simulink model "mcb_pmsm_foc_sensorless_hvkit_f28069m"  (R2021b)
settings: Solver=FixedStepDiscrete  StartTime=0.0  StopTime=8  RelTol=1e-3  EnableMultiTasking=on
InitFcn:
  | mcb_pmsm_foc_sensorless_hvkit_f28069m_datascript;
values from neighbouring files (symbols this model uses):
  acceleration = 20000/PU_System.N_base    [mcb_pmsm_foc_dual_f28379d_datascript.m]    (also in mcb_pmsm_foc_sensorless_dyno_f28379d_datascript.m = 20000/PU_System_motor1.N_base; mcb_pmsm_foc_sensorless_f280049C_datascript.m; mcb_pmsm_foc_sensorless_f28027LaunchPad_data.m; mcb_pmsm_foc_sensorless_f28035_datascript.m)
  inverter = mcb_SetInverterParameters('BoostXL-DRV8305')    [mcb_pmsm_foc_dual_f28379d_data.m]    (also in mcb_pmsm_foc_dual_f28379d_datascript.m; mcb_pmsm_foc_f280049C_data.m; mcb_pmsm_foc_f28335_data.m = mcb_SetInverterParameters('DRV8312-C2-KIT'); mcb_pmsm_foc_hall_f28035_data.m = mcb_SetInverterParameters('DRV8312-C2-KIT'))
  PI_params = mcb.internal.SetControllerParameters(pmsm,inverter,PU_System,T_pwm,2*Ts,Ts_speed)    [mcb_pmsm_foc_dual_f28379d_data.m]    (also in mcb_pmsm_foc_dual_f28379d_datascript.m; mcb_pmsm_foc_f280049C_data.m = mcb.internal.SetControllerParameters(pmsm,inverter,PU_System; mcb_pmsm_foc_f28335_data.m = mcb.internal.SetControllerParameters(pmsm,inverter,PU_System; mcb_pmsm_foc_hall_f28035_data.m = mcb.internal.SetControllerParameters(pmsm,inverter,PU_System)
  pmsm = struct    [c28335_pmsmfoc_data.m]    (also in mcb_pmsm_foc_dual_f28379d_data.m = mcb_SetPMSMMotorParameters('Teknic2310P'); mcb_pmsm_foc_dual_f28379d_datascript.m = mcb_SetPMSMMotorParameters('Teknic2310P'); mcb_pmsm_foc_f280049C_data.m = mcb_SetPMSMMotorParameters('BLY171D'); mcb_pmsm_foc_f28335_data.m = mcb_SetPMSMMotorParameters('BLY171D'))
  PWM_frequency = 20e3    (= 20000)    [c28027pmsmfoc_data.m]    (also in c28035pmsmfoc_data.m; c28035pmsmfoc_data_cla.m = 12000; c28069pmsmfoc_data.m; mcb_c2000_open_loop_control_data.m = eval(get_param([bdroot '/Open Loop Control/Parameters/PWM Fr)
  Speed_openLoop_PU = 0.1    [mcb_pmsm_foc_dual_f28379d_data.m]    (also in mcb_pmsm_foc_dual_f28379d_datascript.m; mcb_pmsm_foc_sensorless_dyno_f28379d_data.m; mcb_pmsm_foc_sensorless_dyno_f28379d_datascript.m; mcb_pmsm_foc_sensorless_f280049C_data.m)
  T_Ref_openLoop = 1    [mcb_pmsm_foc_dual_f28379d_data.m]    (also in mcb_pmsm_foc_dual_f28379d_datascript.m; mcb_pmsm_foc_sensorless_dyno_f28379d_data.m; mcb_pmsm_foc_sensorless_dyno_f28379d_datascript.m; mcb_pmsm_foc_sensorless_f280049C_data.m)
  target = mcb_SetProcessorDetails('F28379D',PWM_frequency)    [mcb_pmsm_foc_dual_f28379d_data.m]    (also in mcb_pmsm_foc_dual_f28379d_datascript.m; mcb_pmsm_foc_f280049C_data.m = mcb_SetProcessorDetails('F280049C',PWM_frequency); mcb_pmsm_foc_f28335_data.m = mcb_SetProcessorDetails('F28335',PWM_frequency); mcb_pmsm_foc_hall_f28035_data.m = mcb_SetProcessorDetails('F28035',PWM_frequency))
  Ts_motor = T_pwm/2    (= 2.5e-05)    [mcb_pmsm_foc_dual_f28379d_data.m]    (also in mcb_pmsm_foc_dual_f28379d_datascript.m; mcb_pmsm_foc_f280049C_data.m; mcb_pmsm_foc_f28335_data.m; mcb_pmsm_foc_hall_f28035_data.m)
  Ts_simulink = T_pwm/2    (= 2.5e-05)    [mcb_pmsm_foc_dual_f28379d_data.m]    (also in mcb_pmsm_foc_dual_f28379d_datascript.m; mcb_pmsm_foc_f280049C_data.m; mcb_pmsm_foc_f28335_data.m; mcb_pmsm_foc_hall_f28035_data.m)
  Ts_speed = 20*Ts    (= 0.001)    [mcb_pmsm_foc_dual_f28379d_data.m]    (also in mcb_pmsm_foc_dual_f28379d_datascript.m; mcb_pmsm_foc_f280049C_data.m = 0.0005; mcb_pmsm_foc_f28335_data.m = 0.0005; mcb_pmsm_foc_hall_f28035_data.m = 0.0005)
undefined symbols (not defined in the file or in its folder): Down, GPTRIP1SEL, GPTRIP2SEL, TZ1, TZ2, Up
libraries: c2802xlib x5, c2806xlib x3, demo_controls x1, mcbplantlib x1, mcbcontrolslib x1, mcbpositiondecoderlib x1, autolibpmsmexterior x1
settings Model: ExtModeTrigDuration=8  Creator=The MathWorks, Inc.  LastModifiedBy=The MathWorks, Inc.
settings SolverCC: AlgebraicLoopSolver=TrustRegion
settings DataIOCC: LimitDataPoints=on  SaveFormat=Array  SaveOutput=off  SaveTime=off  ReturnWorkspaceOutputs=off
settings OptimizationCC: DefaultParameterBehavior=Inlined  OptimizeBlockIOStorage=off  BufferReuse=off  GlobalBufferReuse=off  ExpressionFolding=off  ExpressionDepthLimit=2147483647  LocalBlockOutputs=off  InitFltsAndDblsToZero=on  NoFixptDivByZeroProtection=on  EfficientFloat2IntCast=on  EfficientMapNaN2IntZero=off  LifeSpan=inf  MaxStackSize=768  OptimizeDataStoreBuffers=off  BusAssignmentInplaceUpdate=off  EfficientTunableParamExpr=on
settings DebuggingCC: ReadBeforeWriteMsg=DisableAll  WriteAfterWriteMsg=DisableAll  WriteAfterReadMsg=DisableAll  AlgebraicLoopMsg=error  ArtificialAlgebraicLoopMsg=error  CheckSSInitialOutputMsg=off  MergeDetectMultiDrivingBlocksExec=none  SignalResolutionControl=TryResolveAllWithWarning  SolverPrmCheckMsg=warning  InheritedTsInSrcMsg=none  MultiTaskDSMMsg=none  MultiTaskCondExecSysMsg=none  TasksWithSamePriorityMsg=none  SigSpecEnsureSampleTimeMsg=none  IntegerOverflowMsg=none  ParameterPrecisionLossMsg=none  FcnCallInpInsideContextMsg=warning  AllowSymbolicDim=off  StateNameClashWarn=warning  SFUnexpectedBacktrackingDiag=warning  SFNoUnconditionalDefaultTransitionDiag=warning  SFExecutionAtInitializationDiag=none  SFMachineParentedDataDiag=warning  IntegerSaturationMsg=none  ArithmeticOperatorsInVariantConditions=warning
settings HardwareCC: ProdBitPerChar=16  ProdBitPerInt=16  ProdBitPerPointer=32  ProdBitPerSizeT=32  ProdBitPerPtrDiffT=32  ProdLargestAtomicInteger=Integer  ProdLargestAtomicFloat=None  ProdWordSize=16  ProdLongLongMode=on  ProdHWDeviceType=Texas Instruments->C2000  TargetBitPerChar=16  TargetBitPerInt=16  TargetBitPerPointer=16  TargetLargestAtomicInteger=Integer  TargetIntDivRoundTo=Zero  TargetEndianess=LittleEndian  TargetWordSize=16  TargetHWDeviceType=Texas Instruments->C2000
settings ModelReferenceCC: PropagateSignalLabelsOutOfModel=off
settings SFSimCC: SimUseLocalCustomCode=off  MATLABDynamicMemAlloc=off
settings RTWCC: Description=Embedded Coder  SystemTargetFile=ert.tlc  HardwareBoard=TI Piccolo F2806x  TemplateMakefile=ert_default_tmf  PostCodeGenCommand=; codertarget.postCodeGenHookCommand(h)  GenerateReport=on  RTWUseLocalCustomCode=off  Toolchain=Texas Instruments Code Composer Studio (C2000)  BuildConfiguration=Faster Runs  IncludeHyperlinkInReport=on  LaunchReport=on  GenerateTraceInfo=on  GenerateTraceReport=on  GenerateTraceReportSl=on  GenerateTraceReportSf=on  GenerateTraceReportEml=on
settings CodeAppCC: IgnoreCustomStorageClasses=off  CustomSymbolStrType=$N$R$M  StateflowObjectComments=on  InternalIdentifier=Classic
settings ERTTargetCC: TargetFcnLib=ansi_tfl_tmw_new.mat  CodeReplacementLibrary=TI C28x  MultiwordLength=2048  ParMdlRefBuildCompliant=off  CompOptLevelCompliant=off  ConcurrentExecutionCompliant=off  CPPClassGenCompliant=off  ExtModeStaticAllocSize=2048  ExtModeMexFile=TIC2000ExternalModeOpen  ExtModeIntrfLevel=Level2 - Open  InlinedParameterPlacement=NonHierarchical  ConvertIfToSwitch=off  SuppressUnreachableDefaultCases=off  MemSecPackage=tic2000demospkg
settings ConfigComp: CovMetricSettings=dw  CovSaveCumulativeToWorkspaceVar=on  CovSaveSingleToWorkspaceVar=on  CovExternalEMLEnable=off  CovSFcnEnable=off

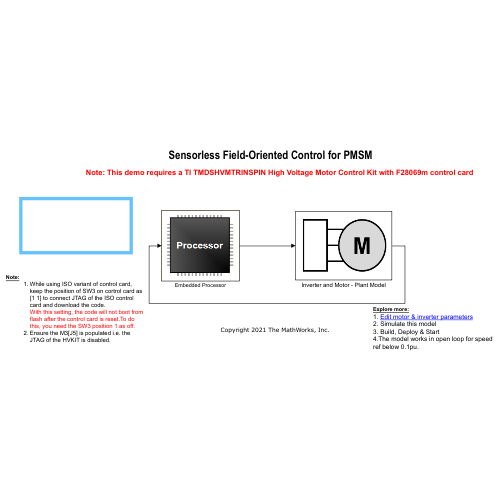
[thumbnail: Simulink's stored preview of the top-level diagram]
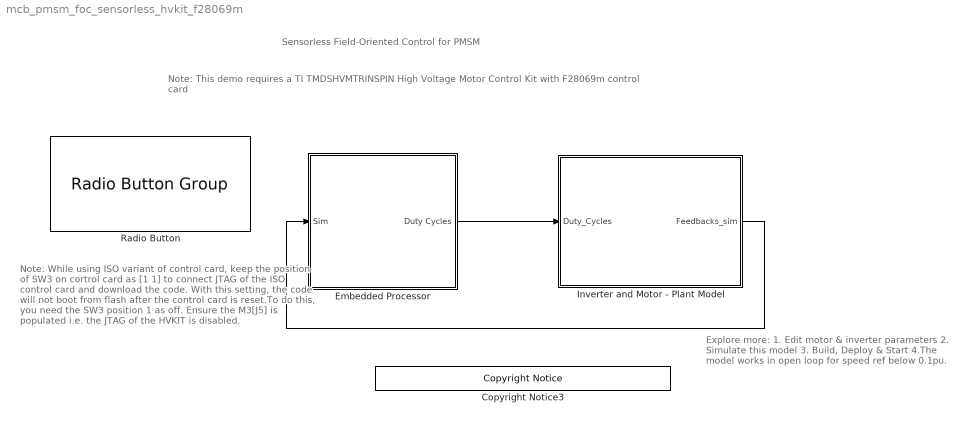
== system mcb_pmsm_foc_sensorless_hvkit_f28069m ==
  note: Sensorless Field-Oriented Control for PMSM
  note: Explore more:
      | 1. Edit motor & inverter parameters
      | 2. Simulate this model
      | 3. Build, Deploy & Start
      | 4.The model works in open loop for speed ref below 0.1pu.
  note: Note: This demo requires a TI TMDSHVMTRINSPIN High Voltage Motor Control Kit with F28069m control card
  note: Note:
      | While using ISO variant of control card, keep the position of SW3 on cortrol card as [1 1] to connect JTAG of the ISO control card and download the code.
      | With this setting, the code will not boot from flash after the control card is reset.To do this, you need the SW3 position 1 as off.
      | Ensure the M3[J5] is populated i.e. the JTAG of the HVKIT is disabled.
  Copyright Notice3 : demo_controls/Copyright Notice  year=2021  prod=tic2000
      settings: SourceProductBaseCode=ME
  Embedded Processor : Subsystem
      mask Display: image('mcb_pmsmfoc_processor.png')
  Inverter and Motor - Plant Model : Subsystem
      mask Display: image('mcb_pmsmfoc_motor.png')
  Radio Button : RadioButtonGroup  LabelPosition=Hide  SelectedLabel=Flux observer  ButtonGroupName=Postion Estimator
      settings: Values={{'Sliding mode observer', 'Flux observer'}, [0 1]}
  wires:
  Embedded Processor/1(Duty Cycles) -> Inverter and Motor - Plant Model/1(Duty_Cycles)
  Inverter and Motor - Plant Model/1(Feedbacks_sim) -> Embedded Processor/1(Sim)

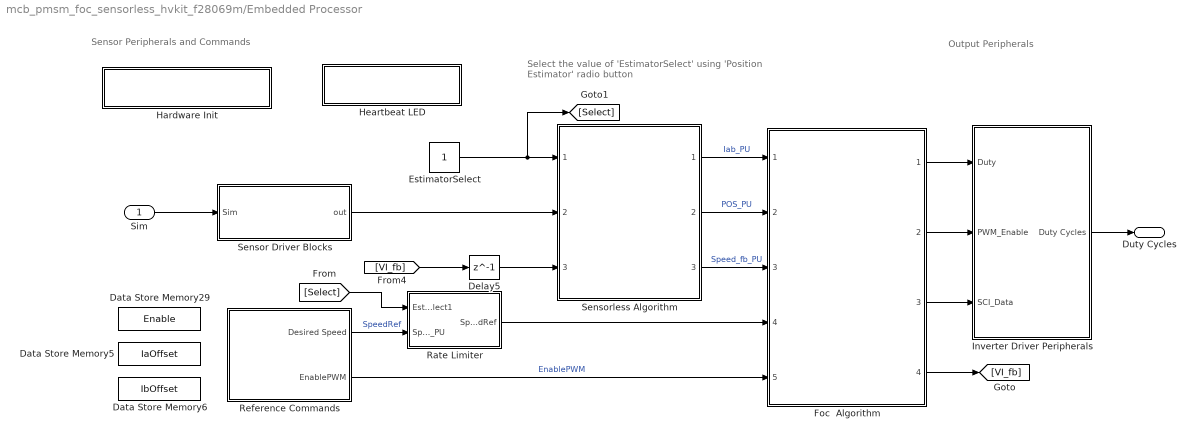
== system mcb_pmsm_foc_sensorless_hvkit_f28069m/Embedded Processor ==
  note: Output Peripherals
  note: Sensor Peripherals and Commands
  note: Select the value of 'EstimatorSelect' using 'Position Estimator' radio button
  Sim : Inport
  Data Store Memory29 : DataStoreMemory  DataStoreName=Enable  ReadBeforeWriteMsg=warning  WriteAfterWriteMsg=warning  WriteAfterReadMsg=warning  InitialValue=1  ShowAdditionalParam=off  OutDataTypeStr=boolean
  Data Store Memory5 : DataStoreMemory  DataStoreName=IaOffset  InitialValue=inverter.CtSensAOffset  ShowAdditionalParam=off  OutDataTypeStr=uint16
  Data Store Memory6 : DataStoreMemory  DataStoreName=IbOffset  InitialValue=inverter.CtSensBOffset  ShowAdditionalParam=off  OutDataTypeStr=uint16
  Delay5 : Delay  DelayLength=1
  EstimatorSelect : Constant
  Foc  Algorithm : Subsystem  ReferencedSubsystem=foc_sensorless_algorithm
  Hardware Init : Subsystem  TreatAsAtomicUnit=on
  Heartbeat LED : Subsystem  TreatAsAtomicUnit=on
  Inverter Driver Peripherals : Subsystem  TreatAsAtomicUnit=on
      settings: RTWSystemCode=Nonreusable function
  Rate Limiter : Subsystem  SystemSampleTime=Ts_speed
  Reference Commands : Subsystem  SystemSampleTime=1e-3
  Sensor Driver Blocks : Subsystem  Variant=on  VariantControlMode=sim codegen switching
  Sensorless Algorithm : Subsystem  TreatAsAtomicUnit=on  ReferencedSubsystem=sensorless_algorithm
      settings: RTWSystemCode=Nonreusable function
  Duty Cycles : Outport
  wires:
  Reference Commands/1(Desired Speed) -> Rate Limiter/2(Speed_Ref_PU)  "SpeedRef"
  Inverter Driver Peripherals/1(Duty Cycles) -> Duty Cycles/1
  Reference Commands/2(EnablePWM) -> Foc  Algorithm/5  "EnablePWM"
  Foc  Algorithm/4 -> [VI_fb]
  [VI_fb] -> Delay5/1
  Foc  Algorithm/3 -> Inverter Driver Peripherals/3(SCI_Data)
  Sensorless Algorithm/1 -> Foc  Algorithm/1  "Iab_PU"
  Sensorless Algorithm/2 -> Foc  Algorithm/2  "POS_PU"
  Sensorless Algorithm/3 -> Foc  Algorithm/3  "Speed_fb_PU"
  Foc  Algorithm/2 -> Inverter Driver Peripherals/2(PWM_Enable)
  Foc  Algorithm/1 -> Inverter Driver Peripherals/1(Duty)
  Sim/1 -> Sensor Driver Blocks/1(Sim)
  Delay5/1 -> Sensorless Algorithm/3
  Sensor Driver Blocks/1(out) -> Sensorless Algorithm/2
  Rate Limiter/1(SpeedRef) -> Foc  Algorithm/4
  EstimatorSelect/1 -> [Select], Sensorless Algorithm/1
  [Select] -> Rate Limiter/1(EstimatorSelect1)

== system mcb_pmsm_foc_sensorless_hvkit_f28069m/Inverter and Motor - Plant Model ==
  Duty_Cycles : Inport
  Inverter and Motor - Plant Model : Subsystem
  RT3 : RateTransition  Deterministic=off
  Rate Transition2 : RateTransition  Deterministic=off  OutPortSampleTime=Ts
  Feedbacks_sim : Outport  VectorParamsAs1DForOutWhenUnconnected=off
  wires:
  RT3/1 -> Inverter and Motor - Plant Model/1(Duty_Cycles)
  Inverter and Motor - Plant Model/1(Feedbacks_sim) -> Rate Transition2/1
  Duty_Cycles/1 -> RT3/1
  Rate Transition2/1 -> Feedbacks_sim/1

== system mcb_pmsm_foc_sensorless_hvkit_f28069m/Embedded Processor/Hardware Init ==
  Event Listener : EventListener  DisableCoverage=on  EventName=reset
  Offset Calculation : Subsystem  Variant=on  VariantControlMode=sim codegen switching  VariantControl=Choice

== system mcb_pmsm_foc_sensorless_hvkit_f28069m/Embedded Processor/Heartbeat LED ==
  note: Heartbeat LED 1HZ
  LED BLINK : Subsystem  Variant=on  VariantControlMode=sim codegen switching  VariantControl=Choice
  RED_LED : Constant  OutDataTypeStr=uint16  SampleTime=0.5
  wires:
  RED_LED/1 -> LED BLINK/1(In1)

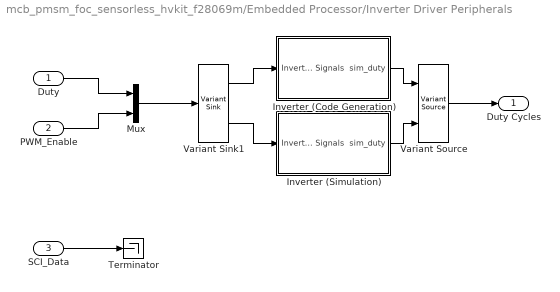
== system mcb_pmsm_foc_sensorless_hvkit_f28069m/Embedded Processor/Inverter Driver Peripherals ==
  Duty : Inport
  PWM_Enable : Inport  Port=2
  SCI_Data : Inport  Port=3
  Inverter (Code Generation) : Subsystem  VariantControl=Choice
  Inverter (Simulation) : Subsystem  VariantControl=(sim)
  Mux : Mux  Inputs=2
  Terminator : Terminator
  Variant Sink1 : VariantSink  VariantControlMode=sim codegen switching
  Variant Source : VariantSource  VariantControlMode=sim codegen switching
  Duty Cycles : Outport  InitialOutput=0  VectorParamsAs1DForOutWhenUnconnected=off
  wires:
  Variant Source/1 -> Duty Cycles/1
  PWM_Enable/1 -> Mux/2
  Duty/1 -> Mux/1
  Mux/1 -> Variant Sink1/1
  Variant Sink1/1 -> Inverter (Code Generation)/1(Inverter Signals)
  Variant Sink1/2 -> Inverter (Simulation)/1(Inverter Signals)
  Inverter (Code Generation)/1(sim_duty) -> Variant Source/1
  Inverter (Simulation)/1(sim_duty) -> Variant Source/2
  SCI_Data/1 -> Terminator/1

== system mcb_pmsm_foc_sensorless_hvkit_f28069m/Embedded Processor/Rate Limiter ==
  EstimatorSelect1 : Inport
  Speed_Ref_PU : Inport  Port=2
  RT3 : RateTransition  Deterministic=off  OutPortSampleTime=Ts_speed
  Slew Rate : Subsystem  TreatAsAtomicUnit=on  SystemSampleTime=Ts_speed
  SpeedRef : Outport
  wires:
  Speed_Ref_PU/1 -> RT3/1
  EstimatorSelect1/1 -> Slew Rate/1(In1)
  RT3/1 -> Slew Rate/2(Speed_Ref)
  Slew Rate/1(Out1) -> SpeedRef/1

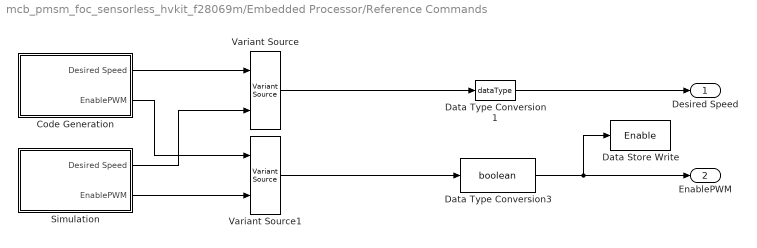
== system mcb_pmsm_foc_sensorless_hvkit_f28069m/Embedded Processor/Reference Commands ==
  Code Generation : Subsystem
  Data Store Write : DataStoreWrite  DataStoreName=Enable  IndexOptions=Index vector (dialog)  Indices=1  OutputSizes=1
  Data Type Conversion1 : DataTypeConversion  OutDataTypeStr=dataType  RndMeth=Simplest
  Data Type Conversion3 : DataTypeConversion  OutDataTypeStr=boolean  RndMeth=Simplest
  Simulation : Subsystem
  Variant Source : VariantSource  VariantControlMode=sim codegen switching
  Variant Source1 : VariantSource  VariantControlMode=sim codegen switching
  Desired Speed : Outport  VectorParamsAs1DForOutWhenUnconnected=off
  EnablePWM : Outport  Port=2
  wires:
  Data Type Conversion3/1 -> Data Store Write/1, EnablePWM/1
  Data Type Conversion1/1 -> Desired Speed/1
  Simulation/2(EnablePWM) -> Variant Source1/2
  Code Generation/2(EnablePWM) -> Variant Source1/1
  Simulation/1(Desired Speed) -> Variant Source/2
  Variant Source1/1 -> Data Type Conversion3/1
  Code Generation/1(Desired Speed) -> Variant Source/1
  Variant Source/1 -> Data Type Conversion1/1

== system mcb_pmsm_foc_sensorless_hvkit_f28069m/Embedded Processor/Sensor Driver Blocks ==
  Sim : Inport
  Sensor Driver Blocks (codegen) : Subsystem  TreatAsAtomicUnit=on  VariantControl=(codegen)
      settings: RTWSystemCode=Nonreusable function
  Sensor Driver Blocks (sim) : Subsystem  VariantControl=(sim)
  out : Outport

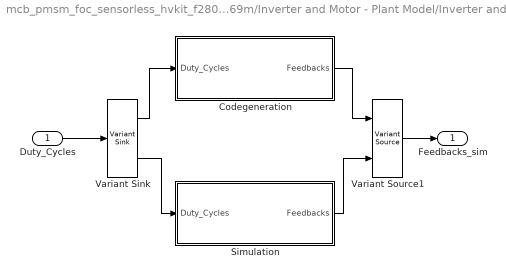
== system mcb_pmsm_foc_sensorless_hvkit_f28069m/Inverter and Motor - Plant Model/Inverter and Motor - Plant Model ==
  Duty_Cycles : Inport
  Codegeneration : Subsystem
  Simulation : Subsystem
  Variant Sink : VariantSink  VariantControlMode=sim codegen switching
  Variant Source1 : VariantSource  VariantControlMode=sim codegen switching
  Feedbacks_sim : Outport  VectorParamsAs1DForOutWhenUnconnected=off
  wires:
  Duty_Cycles/1 -> Variant Sink/1
  Simulation/1(Feedbacks) -> Variant Source1/2
  Variant Sink/2 -> Simulation/1(Duty_Cycles)
  Variant Source1/1 -> Feedbacks_sim/1
  Variant Sink/1 -> Codegeneration/1(Duty_Cycles)
  Codegeneration/1(Feedbacks) -> Variant Source1/1

== system mcb_pmsm_foc_sensorless_hvkit_f28069m/Embedded Processor/Hardware Init/Offset Calculation ==
  Code Generation : Subsystem  VariantControl=(codegen)
  Simulation : Subsystem  VariantControl=(sim)

== system mcb_pmsm_foc_sensorless_hvkit_f28069m/Embedded Processor/Heartbeat LED/LED BLINK ==
  In1 : Inport
  Code generation : Subsystem  VariantControl=(codegen)
  Simulation : Subsystem  VariantControl=(sim)

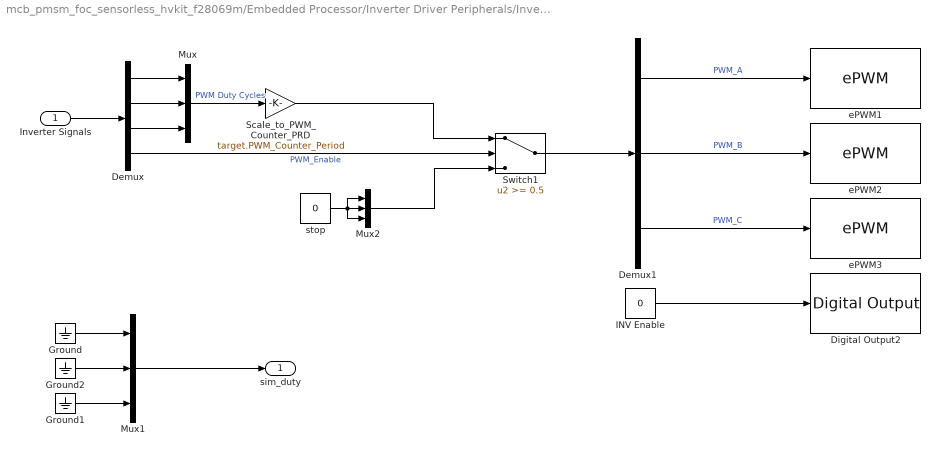
== system mcb_pmsm_foc_sensorless_hvkit_f28069m/Embedded Processor/Inverter Driver Peripherals/Inverter (Code Generation) ==
  Inverter Signals : Inport
  Demux : Demux
  Demux1 : Demux  Outputs=3
  Digital Output2 : c2806xlib/Digital Output  GPIO_Number=GPIO8~GPIO15  GPIO_Bit0=off  GPIO_BIT0_Toggle=off  GPIO_Bit1=off  GPIO_BIT1_Toggle=off  GPIO_Bit2=off  GPIO_BIT2_Toggle=off  GPIO_Bit3=off  GPIO_BIT3_Toggle=off  GPIO_Bit4=off  GPIO_BIT4_Toggle=off  GPIO_Bit5=off  GPIO_BIT5_Toggle=off  GPIO_Bit6=off  GPIO_BIT6_Toggle=off  GPIO_Bit7=on  GPIO_BIT7_Toggle=off
      settings: SourceProductBaseCode=TIC2000
  Ground : Ground
  Ground1 : Ground
  Ground2 : Ground
  INV Enable : Constant  Value=0  OutDataTypeStr=uint16
  Mux : Mux  Inputs=3
  Mux1 : Mux  Inputs=3
  Mux2 : Mux  Inputs=3
  Scale_to_PWM_Counter_PRD : Gain  Gain=target.PWM_Counter_Period  OutDataTypeStr=uint16  RndMeth=Simplest
  Switch1 : Switch  Threshold=0.5
  ePWM1 : c2802xlib/ePWM  PwmType=C2000  useModule=ePWM1  ePWMxLINKTBPRD=Not Linked  periodUnits=Clock cycles  timerSource=Specify via dialog  timerPeriod_clk=target.PWM_Counter_Period+1  timerPeriod_sec=64000  tbshadow=Counter equals to zero  countingMode=Up-Down  phaseActiveEnable=Disable  phaseDirection=Count down after sync  phaseActive=0  synchronizationEnable=off  dcaevt1Sync=off  dcbevt1Sync=off  synchronizationOption=Counter equals to zero (CTR=Zero)  perSynchronizationOption=Counter equals to period (CTR=PRD)  clockPrescale=1  HSclockPrescale=1  enswap=off  ePWMxAStatus=on  ePWMxAactionLogic1=Do nothing  ePWMxAactionLogic2=Do nothing  ePWMxAactionLogic3=Clear  ePWMxAactionLogic4=Set  ePWMxAactionLogic5=Do nothing  ePWMxAactionLogic6=Do nothing  ePWMxACSFenable=off  ePWMxACSFvalue=Forcing disable  ePWMxASFreload=Zero  ePWMxBStatus=off  ePWMxBactionLogic1=Do nothing  ePWMxBactionLogic2=Set  ePWMxBactionLogic3=Do nothing  ePWMxBactionLogic4=Do nothing  ePWMxBactionLogic5=Clear  ePWMxBactionLogic6=Do nothing  ePWMxBCSFenable=off  ePWMxBCSFvalue=Forcing disable  ePWMxBSFreload=Zero  ePWNxBOutWay=off  ePWMxLINKCMPA=Not Linked  CMPAUnits=Clock cycles  CMPASource=Input port  CMPAValue_per=32000  CMPAValue_clk=floor(target.PWM_Counter_Period/2+1)  enCMPAshadow=Counter equals to zero (CTR=Zero)  ePWMxLINKCMPB=Not Linked  CMPBUnits=Clock cycles  CMPBSource=Specify via dialog  CMPBValue_per=50  CMPBValue_clk=floor(target.PWM_Counter_Period/2+1)  enCMPBshadow=Counter equals to zero (CTR=Zero)  ePWMxLINKCMPC=Not Linked  CMPCUnits=Clock cycles  CMPCSource=Specify via dialog  CMPCValue_per=50  CMPCValue_clk=32000  enCMPCshadow=Counter equals to zero (CTR=Zero)  ePWMxLINKCMPD=Not Linked  CMPDUnits=Clock cycles  CMPDSource=Specify via dialog  CMPDValue_per=50  CMPDValue_clk=32000  enCMPDshadow=Counter equals to zero (CTR=Zero)  enableDBePWMxA=on  enableDBePWMxB=on  enhalfcycle=off  DBpolarity=Active high complementary (AHC)  DBedgeDelay=Positive  DBSource_ePWMxA=ePWMxA  DBSource_ePWMxB=ePWMxA  DBPeriodUnits=Clock cycles  DBperiodSource=Specify via dialog  REDperiod=15  FEDperiod=15  REDperiod_sec=0  FEDperiod_sec=0  LoadModeDBRED=Immediate without using shadow  LoadModeDBFED=Immediate without using shadow  adcstartModuleA=on  adcrequestEventA=First event  adcstartEventA=Counter equals to period (CTR=PRD)  adcstartEventA_type2=Digital Compare Module A Event 1 start of conversion (DCAEVT1.soc)  adcstartModuleB=off  adcrequestEventB=First event  adcstartEventB=Counter equals to zero (CTR=Zero)  adcstartEventB_type2=Counter equals to zero (CTR=Zero)  intEn=off  intPrd=First event  intSel=Counter equals to zero (CTR=Zero)  intSel_type2=Counter equals to zero (CTR=Zero)  hrpe=off  enHRPWM=off  HRPWM_LoadMode=Counter equals to period (CTR=PRD)  HRPWM_CTLMode=Duty or Period control mode  HRPWM_EDGMode=Both edge  hrpeb=off  enHRPWMB=off  HRPWM_LoadModeB=Counter equals to zero (CTR=ZERO)  HRPWM_CTLModeB=Duty or Period control mode  HRPWM_EDGModeB=Both edge  enHRDBRED=off  enHRDBFED=off  enSFO=on  enautoconv=on  chopperEnable=off  chopperFrequency=1  chopperFirstwidth=1  chopperDuty=12.5%  tripZonesource=Specify via dialog  tzselOSHT1=off  tzselOSHT2=off  tzselOSHT3=off  tzselOSHDCAEV1=off  tzselOSHDCBEV1=off  tzselCBC1=off  tzselCBC2=off  tzselCBC3=off  tzselCBCDCAEV2=off  tzselCBCDCBEV2=off  tzselOSHT4=off  tzselOSHT5=off  tzselOSHT6=off  tzselCBC4=off  tzselCBC5=off  tzselCBC6=off  enTzOstIntr=off  enTzCbcIntr=off  enTzDCAEVT1Intr=off  enTzDCAEVT2Intr=off  enTzDCBEVT1Intr=off  enTzDCBEVT2Intr=off  ePWMxAforced=No action  ePWMxBforced=No action  DCAEVT1forced=No action  DCBEVT1forced=No action  DCAEVT2forced=No action  DCBEVT2forced=No action  dcah=Trip Zone 1 input (TZ1)  dcal=Trip Zone 2 input (TZ2)  dcbh=Trip Zone 1 input (TZ1)  dcbl=Trip Zone 2 input (TZ2)  dcah_type2=GPTRIP1SEL/(TZ1)  dcal_type2=GPTRIP2SEL/(TZ2)  dcbh_type2=GPTRIP1SEL/(TZ1)  dcbl_type2=GPTRIP2SEL/(TZ2)  gendcaevt1=Event disabled  gendcaevt2=Event disabled  gendcbevt1=Event disabled  gendcbevt2=Event disabled  dcaevt1src=DCAEVT1 with sync  dcaevt2src=DCAEVT2 with sync  dcbevt1src=DCBEVT1 with sync  dcbevt2src=DCBEVT2 with sync  pulsesel=Counter equals to zero (CTR=Zero)  blankinv=off  blankoffset=0  blankwidth=0  evsrcsel=Filtered version of DCAEVT1 (DCAEVT1FILT)  encape=off
  ePWM2 : c2802xlib/ePWM  PwmType=C2000  useModule=ePWM2  ePWMxLINKTBPRD=Not Linked  periodUnits=Clock cycles  timerSource=Specify via dialog  timerPeriod_clk=target.PWM_Counter_Period+1  timerPeriod_sec=64000  tbshadow=Counter equals to zero  countingMode=Up-Down  phaseActiveEnable=Set counter to phase value specified via dialog  phaseDirection=Count up after sync  phaseActive=0  synchronizationEnable=off  dcaevt1Sync=off  dcbevt1Sync=off  synchronizationOption=Pass through (EPWMxSYNCI or SWFSYNC)  perSynchronizationOption=Counter equals to period (CTR=PRD)  clockPrescale=1  HSclockPrescale=1  enswap=off  ePWMxAStatus=on  ePWMxAactionLogic1=Do nothing  ePWMxAactionLogic2=Do nothing  ePWMxAactionLogic3=Clear  ePWMxAactionLogic4=Set  ePWMxAactionLogic5=Do nothing  ePWMxAactionLogic6=Do nothing  ePWMxACSFenable=off  ePWMxACSFvalue=Forcing disable  ePWMxASFreload=Zero  ePWMxBStatus=off  ePWMxBactionLogic1=Do nothing  ePWMxBactionLogic2=Set  ePWMxBactionLogic3=Do nothing  ePWMxBactionLogic4=Do nothing  ePWMxBactionLogic5=Clear  ePWMxBactionLogic6=Do nothing  ePWMxBCSFenable=off  ePWMxBCSFvalue=Forcing disable  ePWMxBSFreload=Zero  ePWNxBOutWay=off  ePWMxLINKCMPA=Not Linked  CMPAUnits=Clock cycles  CMPASource=Input port  CMPAValue_per=32000  CMPAValue_clk=floor(target.PWM_Counter_Period/2+1)  enCMPAshadow=Counter equals to zero (CTR=Zero)  ePWMxLINKCMPB=Not Linked  CMPBUnits=Clock cycles  CMPBSource=Specify via dialog  CMPBValue_per=50  CMPBValue_clk=floor(target.PWM_Counter_Period/2+1)  enCMPBshadow=Counter equals to zero (CTR=Zero)  ePWMxLINKCMPC=Not Linked  CMPCUnits=Clock cycles  CMPCSource=Specify via dialog  CMPCValue_per=50  CMPCValue_clk=32000  enCMPCshadow=Counter equals to zero (CTR=Zero)  ePWMxLINKCMPD=Not Linked  CMPDUnits=Clock cycles  CMPDSource=Specify via dialog  CMPDValue_per=50  CMPDValue_clk=32000  enCMPDshadow=Counter equals to zero (CTR=Zero)  enableDBePWMxA=on  enableDBePWMxB=on  enhalfcycle=off  DBpolarity=Active high complementary (AHC)  DBedgeDelay=Positive  DBSource_ePWMxA=ePWMxA  DBSource_ePWMxB=ePWMxA  DBPeriodUnits=Clock cycles  DBperiodSource=Specify via dialog  REDperiod=15  FEDperiod=15  REDperiod_sec=0  FEDperiod_sec=0  LoadModeDBRED=Immediate without using shadow  LoadModeDBFED=Immediate without using shadow  adcstartModuleA=off  adcrequestEventA=First event  adcstartEventA=Digital Compare Module A Event 1 start of conversion (DCAEVT1.soc)  adcstartEventA_type2=Digital Compare Module A Event 1 start of conversion (DCAEVT1.soc)  adcstartModuleB=off  adcrequestEventB=First event  adcstartEventB=Counter equals to zero (CTR=Zero)  adcstartEventB_type2=Counter equals to zero (CTR=Zero)  intEn=off  intPrd=First event  intSel=Counter equals to zero (CTR=Zero)  intSel_type2=Counter equals to zero (CTR=Zero)  hrpe=off  enHRPWM=off  HRPWM_LoadMode=Counter equals to period (CTR=PRD)  HRPWM_CTLMode=Duty or Period control mode  HRPWM_EDGMode=Both edge  hrpeb=off  enHRPWMB=off  HRPWM_LoadModeB=Counter equals to zero (CTR=ZERO)  HRPWM_CTLModeB=Duty or Period control mode  HRPWM_EDGModeB=Both edge  enHRDBRED=off  enHRDBFED=off  enSFO=on  enautoconv=on  chopperEnable=off  chopperFrequency=1  chopperFirstwidth=1  chopperDuty=12.5%  tripZonesource=Specify via dialog  tzselOSHT1=off  tzselOSHT2=off  tzselOSHT3=off  tzselOSHDCAEV1=off  tzselOSHDCBEV1=off  tzselCBC1=off  tzselCBC2=off  tzselCBC3=off  tzselCBCDCAEV2=off  tzselCBCDCBEV2=off  tzselOSHT4=off  tzselOSHT5=off  tzselOSHT6=off  tzselCBC4=off  tzselCBC5=off  tzselCBC6=off  enTzOstIntr=off  enTzCbcIntr=off  enTzDCAEVT1Intr=off  enTzDCAEVT2Intr=off  enTzDCBEVT1Intr=off  enTzDCBEVT2Intr=off  ePWMxAforced=No action  ePWMxBforced=No action  DCAEVT1forced=No action  DCBEVT1forced=No action  DCAEVT2forced=No action  DCBEVT2forced=No action  dcah=Trip Zone 1 input (TZ1)  dcal=Trip Zone 2 input (TZ2)  dcbh=Trip Zone 1 input (TZ1)  dcbl=Trip Zone 2 input (TZ2)  dcah_type2=GPTRIP1SEL/(TZ1)  dcal_type2=GPTRIP2SEL/(TZ2)  dcbh_type2=GPTRIP1SEL/(TZ1)  dcbl_type2=GPTRIP2SEL/(TZ2)  gendcaevt1=Event disabled  gendcaevt2=Event disabled  gendcbevt1=Event disabled  gendcbevt2=Event disabled  dcaevt1src=DCAEVT1 with sync  dcaevt2src=DCAEVT2 with sync  dcbevt1src=DCBEVT1 with sync  dcbevt2src=DCBEVT2 with sync  pulsesel=Counter equals to zero (CTR=Zero)  blankinv=off  blankoffset=0  blankwidth=0  evsrcsel=Filtered version of DCAEVT1 (DCAEVT1FILT)  encape=off
  ePWM3 : c2802xlib/ePWM  PwmType=C2000  useModule=ePWM3  ePWMxLINKTBPRD=Not Linked  periodUnits=Clock cycles  timerSource=Specify via dialog  timerPeriod_clk=target.PWM_Counter_Period+1  timerPeriod_sec=64000  tbshadow=Counter equals to zero  countingMode=Up-Down  phaseActiveEnable=Set counter to phase value specified via dialog  phaseDirection=Count up after sync  phaseActive=0  synchronizationEnable=off  dcaevt1Sync=off  dcbevt1Sync=off  synchronizationOption=Disable  perSynchronizationOption=Counter equals to period (CTR=PRD)  clockPrescale=1  HSclockPrescale=1  enswap=off  ePWMxAStatus=on  ePWMxAactionLogic1=Do nothing  ePWMxAactionLogic2=Do nothing  ePWMxAactionLogic3=Clear  ePWMxAactionLogic4=Set  ePWMxAactionLogic5=Do nothing  ePWMxAactionLogic6=Do nothing  ePWMxACSFenable=off  ePWMxACSFvalue=Forcing disable  ePWMxASFreload=Zero  ePWMxBStatus=off  ePWMxBactionLogic1=Do nothing  ePWMxBactionLogic2=Set  ePWMxBactionLogic3=Do nothing  ePWMxBactionLogic4=Do nothing  ePWMxBactionLogic5=Clear  ePWMxBactionLogic6=Do nothing  ePWMxBCSFenable=off  ePWMxBCSFvalue=Forcing disable  ePWMxBSFreload=Zero  ePWNxBOutWay=off  ePWMxLINKCMPA=Not Linked  CMPAUnits=Clock cycles  CMPASource=Input port  CMPAValue_per=32000  CMPAValue_clk=floor(target.PWM_Counter_Period/2+1)  enCMPAshadow=Counter equals to zero (CTR=Zero)  ePWMxLINKCMPB=Not Linked  CMPBUnits=Clock cycles  CMPBSource=Specify via dialog  CMPBValue_per=50  CMPBValue_clk=floor(target.PWM_Counter_Period/2+1)  enCMPBshadow=Counter equals to zero (CTR=Zero)  ePWMxLINKCMPC=Not Linked  CMPCUnits=Clock cycles  CMPCSource=Specify via dialog  CMPCValue_per=50  CMPCValue_clk=32000  enCMPCshadow=Counter equals to zero (CTR=Zero)  ePWMxLINKCMPD=Not Linked  CMPDUnits=Clock cycles  CMPDSource=Specify via dialog  CMPDValue_per=50  CMPDValue_clk=32000  enCMPDshadow=Counter equals to zero (CTR=Zero)  enableDBePWMxA=on  enableDBePWMxB=on  enhalfcycle=off  DBpolarity=Active high complementary (AHC)  DBedgeDelay=Positive  DBSource_ePWMxA=ePWMxA  DBSource_ePWMxB=ePWMxA  DBPeriodUnits=Clock cycles  DBperiodSource=Specify via dialog  REDperiod=15  FEDperiod=15  REDperiod_sec=0  FEDperiod_sec=0  LoadModeDBRED=Immediate without using shadow  LoadModeDBFED=Immediate without using shadow  adcstartModuleA=off  adcrequestEventA=First event  adcstartEventA=Digital Compare Module A Event 1 start of conversion (DCAEVT1.soc)  adcstartEventA_type2=Digital Compare Module A Event 1 start of conversion (DCAEVT1.soc)  adcstartModuleB=off  adcrequestEventB=First event  adcstartEventB=Counter equals to zero (CTR=Zero)  adcstartEventB_type2=Counter equals to zero (CTR=Zero)  intEn=off  intPrd=First event  intSel=Counter equals to zero (CTR=Zero)  intSel_type2=Counter equals to zero (CTR=Zero)  hrpe=off  enHRPWM=off  HRPWM_LoadMode=Counter equals to period (CTR=PRD)  HRPWM_CTLMode=Duty or Period control mode  HRPWM_EDGMode=Both edge  hrpeb=off  enHRPWMB=off  HRPWM_LoadModeB=Counter equals to zero (CTR=ZERO)  HRPWM_CTLModeB=Duty or Period control mode  HRPWM_EDGModeB=Both edge  enHRDBRED=off  enHRDBFED=off  enSFO=on  enautoconv=on  chopperEnable=off  chopperFrequency=1  chopperFirstwidth=1  chopperDuty=12.5%  tripZonesource=Specify via dialog  tzselOSHT1=off  tzselOSHT2=off  tzselOSHT3=off  tzselOSHDCAEV1=off  tzselOSHDCBEV1=off  tzselCBC1=off  tzselCBC2=off  tzselCBC3=off  tzselCBCDCAEV2=off  tzselCBCDCBEV2=off  tzselOSHT4=off  tzselOSHT5=off  tzselOSHT6=off  tzselCBC4=off  tzselCBC5=off  tzselCBC6=off  enTzOstIntr=off  enTzCbcIntr=off  enTzDCAEVT1Intr=off  enTzDCAEVT2Intr=off  enTzDCBEVT1Intr=off  enTzDCBEVT2Intr=off  ePWMxAforced=No action  ePWMxBforced=No action  DCAEVT1forced=No action  DCBEVT1forced=No action  DCAEVT2forced=No action  DCBEVT2forced=No action  dcah=Trip Zone 1 input (TZ1)  dcal=Trip Zone 2 input (TZ2)  dcbh=Trip Zone 1 input (TZ1)  dcbl=Trip Zone 2 input (TZ2)  dcah_type2=GPTRIP1SEL/(TZ1)  dcal_type2=GPTRIP2SEL/(TZ2)  dcbh_type2=GPTRIP1SEL/(TZ1)  dcbl_type2=GPTRIP2SEL/(TZ2)  gendcaevt1=Event disabled  gendcaevt2=Event disabled  gendcbevt1=Event disabled  gendcbevt2=Event disabled  dcaevt1src=DCAEVT1 with sync  dcaevt2src=DCAEVT2 with sync  dcbevt1src=DCBEVT1 with sync  dcbevt2src=DCBEVT2 with sync  pulsesel=Counter equals to zero (CTR=Zero)  blankinv=off  blankoffset=0  blankwidth=0  evsrcsel=Filtered version of DCAEVT1 (DCAEVT1FILT)  encape=off
  stop : Constant  Value=0  OutDataTypeStr=uint16
  sim_duty : Outport  VectorParamsAs1DForOutWhenUnconnected=off
  wires:
  Demux1/3 -> ePWM3/1  "PWM_C"
  Scale_to_PWM_Counter_PRD/1 -> Switch1/1
  Mux2/1 -> Switch1/3
  stop/1 -> Mux2/3, Mux2/2, Mux2/1
  Demux/4 -> Switch1/2  "PWM_Enable"
  Inverter Signals/1 -> Demux/1
  Demux1/2 -> ePWM2/1  "PWM_B"
  Switch1/1 -> Demux1/1
  Demux1/1 -> ePWM1/1  "PWM_A"
  Mux/1 -> Scale_to_PWM_Counter_PRD/1  "PWM Duty Cycles"
  Ground/1 -> Mux1/1
  Ground1/1 -> Mux1/3
  Ground2/1 -> Mux1/2
  Mux1/1 -> sim_duty/1
  Demux/1 -> Mux/1
  Demux/2 -> Mux/2
  Demux/3 -> Mux/3
  INV Enable/1 -> Digital Output2/1

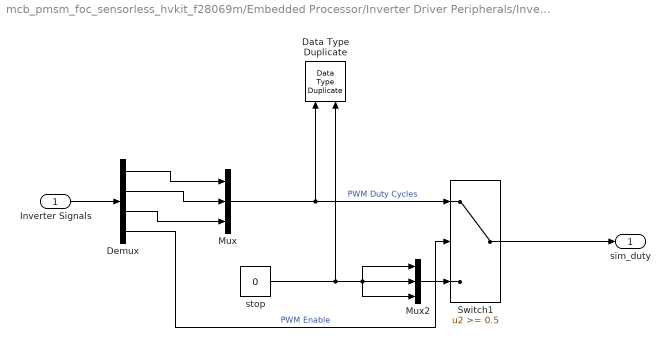
== system mcb_pmsm_foc_sensorless_hvkit_f28069m/Embedded Processor/Inverter Driver Peripherals/Inverter (Simulation) ==
  Inverter Signals : Inport
  Data Type Duplicate : DataTypeDuplicate
  Demux : Demux
  Mux : Mux  Inputs=3
  Mux2 : Mux  Inputs=3
  Switch1 : Switch  Threshold=0.5  RndMeth=Simplest
  stop : Constant  Value=0  OutDataTypeStr=Inherit: Inherit via back propagation
  sim_duty : Outport  VectorParamsAs1DForOutWhenUnconnected=off
  wires:
  stop/1 -> Data Type Duplicate/2, Mux2/1, Mux2/3, Mux2/2
  Mux2/1 -> Switch1/3
  Switch1/1 -> sim_duty/1
  Inverter Signals/1 -> Demux/1
  Demux/4 -> Switch1/2  "PWM Enable"
  Mux/1 -> Data Type Duplicate/1, Switch1/1  "PWM Duty Cycles"
  Demux/1 -> Mux/1
  Demux/2 -> Mux/2
  Demux/3 -> Mux/3

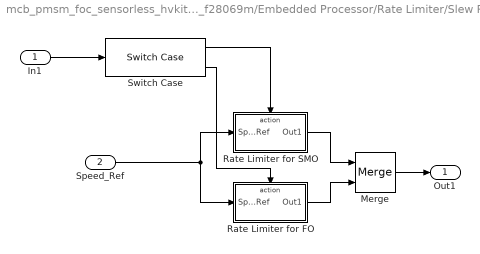
== system mcb_pmsm_foc_sensorless_hvkit_f28069m/Embedded Processor/Rate Limiter/Slew Rate ==
  In1 : Inport
  Speed_Ref : Inport  Port=2
  Merge : Merge
  Rate Limiter for FO : Subsystem  TreatAsAtomicUnit=on
  Rate Limiter for SMO : Subsystem  TreatAsAtomicUnit=on
  Switch Case : SwitchCase  CaseConditions={0,1}  ShowDefaultCase=off
  Out1 : Outport
  wires:
  Switch Case/1 -> Rate Limiter for SMO/Action
  Merge/1 -> Out1/1
  Rate Limiter for FO/1(Out1) -> Merge/2
  Speed_Ref/1 -> Rate Limiter for FO/1(Speed_Ref), Rate Limiter for SMO/1(Speed_Ref)
  Switch Case/2 -> Rate Limiter for FO/Action
  Rate Limiter for SMO/1(Out1) -> Merge/1
  In1/1 -> Switch Case/1

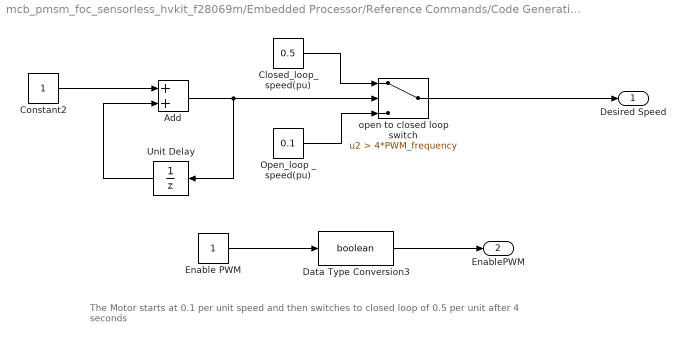
== system mcb_pmsm_foc_sensorless_hvkit_f28069m/Embedded Processor/Reference Commands/Code Generation ==
  note: The Motor starts at 0.1 per unit speed and then switches to closed loop of 0.5 per unit after 4 seconds
  Add : Sum  OutDataTypeStr=uint32
  Closed_loop_speed(pu) : Constant  Value=0.5  OutDataTypeStr=dataType
  Constant2 : Constant  OutDataTypeStr=uint32
  Data Type Conversion3 : DataTypeConversion  OutDataTypeStr=boolean  RndMeth=Simplest
  Enable PWM : Constant  OutDataTypeStr=uint16
  Open_loop _speed(pu) : Constant  Value=0.1  OutDataTypeStr=dataType
  Unit Delay : UnitDelay  SampleTime=-1  HasFrameUpgradeWarning=on
  open to closed loop switch : Switch  Criteria=u2 > Threshold  Threshold=4*PWM_frequency
  Desired Speed : Outport  VectorParamsAs1DForOutWhenUnconnected=off
  EnablePWM : Outport  Port=2
  wires:
  Data Type Conversion3/1 -> EnablePWM/1
  Enable PWM/1 -> Data Type Conversion3/1
  Closed_loop_speed(pu)/1 -> open to closed loop switch/1
  Constant2/1 -> Add/1
  Open_loop _speed(pu)/1 -> open to closed loop switch/3
  Unit Delay/1 -> Add/2
  Add/1 -> Unit Delay/1, open to closed loop switch/2
  open to closed loop switch/1 -> Desired Speed/1

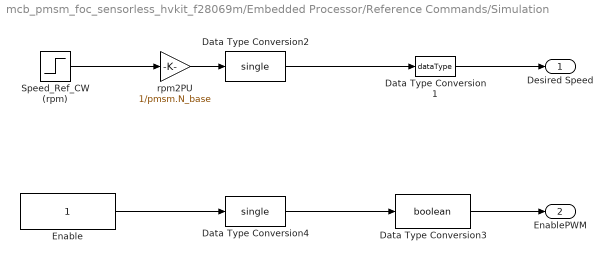
== system mcb_pmsm_foc_sensorless_hvkit_f28069m/Embedded Processor/Reference Commands/Simulation ==
  Data Type Conversion1 : DataTypeConversion  OutDataTypeStr=dataType  RndMeth=Simplest
  Data Type Conversion2 : DataTypeConversion  OutDataTypeStr=single  RndMeth=Simplest
  Data Type Conversion3 : DataTypeConversion  OutDataTypeStr=boolean  RndMeth=Simplest
  Data Type Conversion4 : DataTypeConversion  OutDataTypeStr=single  RndMeth=Simplest
  Enable : Constant  OutDataTypeStr=dataType  SampleTime=-1
  Speed_Ref_CW (rpm) : Step  Time=T_Ref_openLoop  Before=Speed_openLoop_PU*pmsm.N_base  After=0.5*pmsm.N_base
  rpm2PU : Gain  Gain=1/pmsm.N_base  RndMeth=Simplest  OutDataTypeStr=Inherit: Same as input
  Desired Speed : Outport
  EnablePWM : Outport  Port=2
  wires:
  Data Type Conversion2/1 -> Data Type Conversion1/1
  rpm2PU/1 -> Data Type Conversion2/1
  Enable/1 -> Data Type Conversion4/1
  Speed_Ref_CW (rpm)/1 -> rpm2PU/1
  Data Type Conversion4/1 -> Data Type Conversion3/1
  Data Type Conversion1/1 -> Desired Speed/1
  Data Type Conversion3/1 -> EnablePWM/1

== system mcb_pmsm_foc_sensorless_hvkit_f28069m/Embedded Processor/Sensor Driver Blocks/Sensor Driver Blocks (codegen) ==
  Sim : Inport
  IA Measurement : c2802xlib/ADC  blkParamProc=C2000  ADCModule=1  samplingMode=Single sample mode  ADCResolution=12-bit (Single-ended input)  useSOC1=SOC0  useSOC2=SOC0_SOC1  SOCAcquisitionWindow=7  SOCTriggerSource=ePWM1_ADCSOCA  SOCInterruptTrigger=No ADCINT  Ts=-1  dType=uint16  postInterrupt=off  interruptSel=ADCINT1  ADCINTContinuous=on  endma=off  chdma=1  conv1=ADCINB3  conv2=ADCINA1 and ADCINB1  conv1_Type4=ADCIN0  conv2_Type4=ADCIN0 and ADCIN1
  IB Measurement : c2802xlib/ADC  blkParamProc=C2000  ADCModule=1  samplingMode=Single sample mode  ADCResolution=12-bit (Single-ended input)  useSOC1=SOC1  useSOC2=SOC0_SOC1  SOCAcquisitionWindow=7  SOCTriggerSource=ePWM1_ADCSOCA  SOCInterruptTrigger=No ADCINT  Ts=-1  dType=uint16  postInterrupt=on  interruptSel=ADCINT1  ADCINTContinuous=on  endma=off  chdma=1  conv1=ADCINB5  conv2=ADCINA1 and ADCINB1  conv1_Type4=ADCIN0  conv2_Type4=ADCIN0 and ADCIN1
  Mux1 : Mux  Inputs=2
  Terminator : Terminator
  out : Outport
  wires:
  Mux1/1 -> out/1
  Sim/1 -> Terminator/1
  IA Measurement/1 -> Mux1/1
  IB Measurement/1 -> Mux1/2

== system mcb_pmsm_foc_sensorless_hvkit_f28069m/Embedded Processor/Sensor Driver Blocks/Sensor Driver Blocks (sim) ==
  Sim : Inport
  out : Outport
  wires:
  Sim/1 -> out/1

== system mcb_pmsm_foc_sensorless_hvkit_f28069m/Inverter and Motor - Plant Model/Inverter and Motor - Plant Model/Codegeneration ==
  Duty_Cycles : Inport
  Ground : Ground
  Terminator : Terminator
  Feedbacks : Outport  VectorParamsAs1DForOutWhenUnconnected=off
  wires:
  Duty_Cycles/1 -> Terminator/1
  Ground/1 -> Feedbacks/1

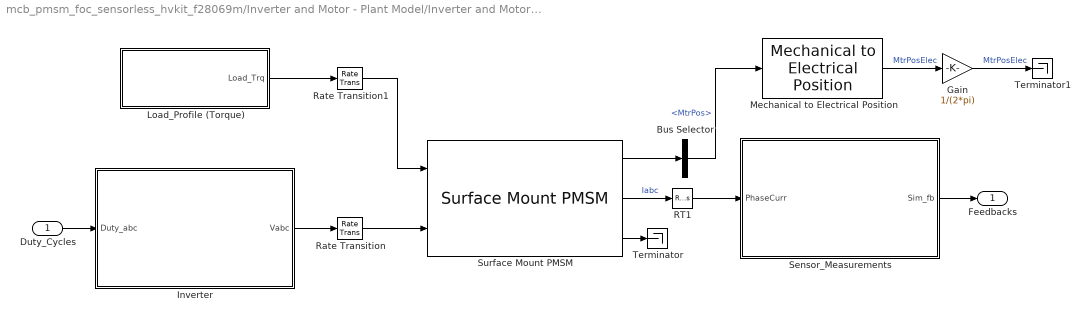
== system mcb_pmsm_foc_sensorless_hvkit_f28069m/Inverter and Motor - Plant Model/Inverter and Motor - Plant Model/Simulation ==
  Duty_Cycles : Inport
  Bus Selector : BusSelector  OutputSignals=MtrPos
  Gain : Gain  Gain=1/(2*pi)  OutDataTypeStr=Inherit: Same as input
  Inverter : Subsystem
  Load_Profile (Torque) : Subsystem
  Mechanical to Electrical Position : mcbpositiondecoderlib/Mechanical to Electrical Position  NrPP=pmsm.p  selectedRange=Radians  MechOfstInputType=Specify via dialog  mechOffsetIn=0  maxAngleIn=2*pi  InputDataType=single  VariantSelect=floating-point
      settings: SourceProductBaseCode=MT
  RT1 : RateTransition  Deterministic=off  OutPortSampleTime=Ts_simulink
  Rate Transition : RateTransition  Deterministic=off  OutPortSampleTime=Ts_motor
  Rate Transition1 : RateTransition  Deterministic=off  OutPortSampleTime=Ts_motor
  Sensor_Measurements : Subsystem
  Surface Mount PMSM : autolibpmsmexterior/Surface Mount PMSM  port_config=Torque  sim_type=Discrete  Ts=Ts_motor  P=pmsm.p  Rs=pmsm.Rs + inverter.R_board  Ldq_=pmsm.Ld  KConstText=Permanent flux linkage constant (lambda_pm):  lambda_pm=pmsm.FluxPM  Ke=159.9771  Kt=1.323  mechanical=[pmsm.J, pmsm.B, 0]  idq0=[0 0]  theta_init=0  omega_init=0  KConst=pmsm.FluxPM  lambda_pm_calc=pmsm.FluxPM  RefBlkName='autolibpmsmexterior/Surface Mount PMSM'  aMode=5  Ldq="[0.0002      0.0002]"
      settings: SourceProductBaseCode=PW,DR,MT,UV,VE
  Terminator : Terminator
  Terminator1 : Terminator
  Feedbacks : Outport  VectorParamsAs1DForOutWhenUnconnected=off
  wires:
  RT1/1 -> Sensor_Measurements/1(PhaseCurr)
  Load_Profile (Torque)/1(Load_Trq) -> Rate Transition1/1
  Surface Mount PMSM/2 -> RT1/1  "Iabc"
  Sensor_Measurements/1(Sim_fb) -> Feedbacks/1
  Gain/1 -> Terminator1/1  "MtrPosElec"
  Inverter/1(Vabc) -> Rate Transition/1
  Surface Mount PMSM/3 -> Terminator/1
  Surface Mount PMSM/1 -> Bus Selector/1
  Mechanical to Electrical Position/1 -> Gain/1  "MtrPosElec"
  Duty_Cycles/1 -> Inverter/1(Duty_abc)
  Rate Transition/1 -> Surface Mount PMSM/2
  Bus Selector/1 -> Mechanical to Electrical Position/1  "<MtrPos>"
  Rate Transition1/1 -> Surface Mount PMSM/1

== system mcb_pmsm_foc_sensorless_hvkit_f28069m/Embedded Processor/Hardware Init/Offset Calculation/Code Generation ==
  DRV Enable : Subsystem  Priority=1
  Default ADC Offset : Subsystem  Priority=1001  TreatAsAtomicUnit=on

== system mcb_pmsm_foc_sensorless_hvkit_f28069m/Embedded Processor/Hardware Init/Offset Calculation/Simulation ==

== system mcb_pmsm_foc_sensorless_hvkit_f28069m/Embedded Processor/Heartbeat LED/LED BLINK/Code generation ==
  note: Heartbeat LED 1HZ
  In1 : Inport
  Digital Output1 : c2806xlib/Digital Output  GPIO_Number=GPIO24~GPIO31  GPIO_Bit0=off  GPIO_BIT0_Toggle=off  GPIO_Bit1=off  GPIO_BIT1_Toggle=off  GPIO_Bit2=off  GPIO_BIT2_Toggle=off  GPIO_Bit3=off  GPIO_BIT3_Toggle=off  GPIO_Bit4=off  GPIO_BIT4_Toggle=off  GPIO_Bit5=off  GPIO_BIT5_Toggle=off  GPIO_Bit6=off  GPIO_BIT6_Toggle=off  GPIO_Bit7=on  GPIO_BIT7_Toggle=on
      settings: SourceProductBaseCode=TIC2000
  wires:
  In1/1 -> Digital Output1/1

== system mcb_pmsm_foc_sensorless_hvkit_f28069m/Embedded Processor/Heartbeat LED/LED BLINK/Simulation ==
  In1 : Inport
  Simulation_Terminator : Terminator
  wires:
  In1/1 -> Simulation_Terminator/1

== system mcb_pmsm_foc_sensorless_hvkit_f28069m/Embedded Processor/Rate Limiter/Slew Rate/Rate Limiter for FO ==
  Speed_Ref : Inport
  Action Port : ActionPort
  Out1 : Outport
  wires:
  Speed_Ref/1 -> Out1/1

== system mcb_pmsm_foc_sensorless_hvkit_f28069m/Embedded Processor/Rate Limiter/Slew Rate/Rate Limiter for SMO ==
  Speed_Ref : Inport
  Action Port : ActionPort
  Rate Limiter : RateLimiter  RisingSlewLimit=acceleration  FallingSlewLimit=-acceleration  SampleTimeMode=inherited  InitialCondition=Speed_openLoop_PU
  Rate Limiter1 : RateLimiter  RisingSlewLimit=acceleration  FallingSlewLimit=-acceleration  SampleTimeMode=inherited  InitialCondition=-Speed_openLoop_PU
  Switch : Switch
  Out1 : Outport
  wires:
  Speed_Ref/1 -> Rate Limiter/1, Rate Limiter1/1, Switch/2
  Switch/1 -> Out1/1
  Rate Limiter1/1 -> Switch/3
  Rate Limiter/1 -> Switch/1

== system mcb_pmsm_foc_sensorless_hvkit_f28069m/Inverter and Motor - Plant Model/Inverter and Motor - Plant Model/Simulation/Inverter ==
  Duty_abc : Inport
  Average-Value Inverter : mcbplantlib/Average-Value Inverter
  Constant2 : Constant  Value=inverter.V_dc  OutDataTypeStr=single  SampleTime=-1
  Data Type Conversion1 : DataTypeConversion  OutDataTypeStr=single  RndMeth=Simplest
  Rate Transition3 : RateTransition  Deterministic=off  OutPortSampleTime=Ts_inverter
  Vabc : Outport  VectorParamsAs1DForOutWhenUnconnected=off
  wires:
  Constant2/1 -> Average-Value Inverter/2
  Data Type Conversion1/1 -> Rate Transition3/1
  Duty_abc/1 -> Data Type Conversion1/1
  Average-Value Inverter/1 -> Vabc/1
  Rate Transition3/1 -> Average-Value Inverter/1

== system mcb_pmsm_foc_sensorless_hvkit_f28069m/Inverter and Motor - Plant Model/Inverter and Motor - Plant Model/Simulation/Load_Profile (Torque) ==
  Data Type Conversion : DataTypeConversion  OutDataTypeStr=single
  IIR Filter : mcbcontrolslib/IIR Filter  VariantControl=Low Pass Filter  VariantSelect=Low-pass  Filter_constant=0.0001  advancedSettings=off  Ts=50e-6  cutOff_freq=0.31834
      settings: SourceProductBaseCode=MT
  T_load : Step  Time=4  Before=0.05*pmsm.T_rated  After=0.5*pmsm.T_rated  SampleTime=Ts_simulink
  Load_Trq : Outport  VectorParamsAs1DForOutWhenUnconnected=off
  wires:
  Data Type Conversion/1 -> IIR Filter/1
  IIR Filter/1 -> Load_Trq/1
  T_load/1 -> Data Type Conversion/1

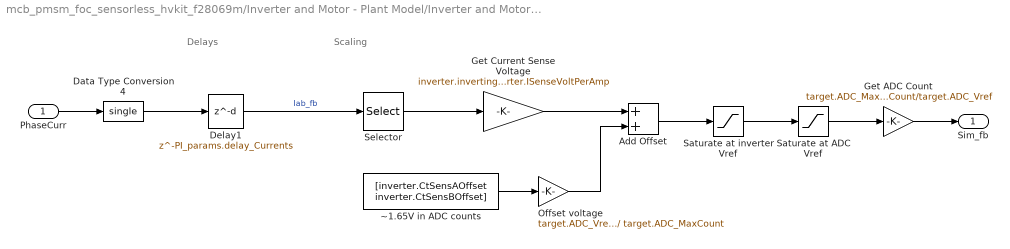
== system mcb_pmsm_foc_sensorless_hvkit_f28069m/Inverter and Motor - Plant Model/Inverter and Motor - Plant Model/Simulation/Sensor_Measurements ==
  note: Scaling
  note: Delays
  PhaseCurr : Inport
  Add Offset : Sum  RndMeth=Simplest
  Data Type Conversion4 : DataTypeConversion  OutDataTypeStr=single  RndMeth=Simplest
  Delay1 : Delay  DelayLength=PI_params.delay_Currents
  Get ADC Count : Gain  Gain=target.ADC_MaxCount/target.ADC_Vref  OutMin=0  OutMax=target.ADC_MaxCount  OutDataTypeStr=uint16  RndMeth=Simplest
  Get Current Sense Voltage : Gain  Gain=inverter.invertingAmp * inverter.ISenseVoltPerAmp  RndMeth=Simplest  OutDataTypeStr=Inherit: Same as input
  Offset voltage : Gain  Gain=target.ADC_Vref / target.ADC_MaxCount  RndMeth=Simplest
  Saturate at ADC Vref : Saturate  UpperLimit=target.ADC_Vref  LowerLimit=0
  Saturate at inverter Vref : Saturate  UpperLimit=inverter.ISenseVref  LowerLimit=0
  Selector : Selector  InputPortWidth=3  IndexOptions=Index vector (dialog)  Indices=[1 2]  OutputSizes=1
  ~1.65V in ADC counts : Constant  Value=[inverter.CtSensAOffset inverter.CtSensBOffset]  OutDataTypeStr=uint16  SampleTime=-1
  Sim_fb : Outport  VectorParamsAs1DForOutWhenUnconnected=off
  wires:
  Delay1/1 -> Selector/1  "Iab_fb"
  Data Type Conversion4/1 -> Delay1/1
  PhaseCurr/1 -> Data Type Conversion4/1
  Add Offset/1 -> Saturate at inverter Vref/1
  Saturate at inverter Vref/1 -> Saturate at ADC Vref/1
  ~1.65V in ADC counts/1 -> Offset voltage/1
  Get Current Sense Voltage/1 -> Add Offset/1
  Saturate at ADC Vref/1 -> Get ADC Count/1
  Selector/1 -> Get Current Sense Voltage/1
  Offset voltage/1 -> Add Offset/2
  Get ADC Count/1 -> Sim_fb/1

== system mcb_pmsm_foc_sensorless_hvkit_f28069m/Embedded Processor/Hardware Init/Offset Calculation/Code Generation/DRV Enable ==
  note: Enable PWM output
  Digital Output1 : c2806xlib/Digital Output  GPIO_Number=GPIO8~GPIO15  GPIO_Bit0=off  GPIO_BIT0_Toggle=off  GPIO_Bit1=off  GPIO_BIT1_Toggle=off  GPIO_Bit2=off  GPIO_BIT2_Toggle=off  GPIO_Bit3=off  GPIO_BIT3_Toggle=off  GPIO_Bit4=off  GPIO_BIT4_Toggle=off  GPIO_Bit5=off  GPIO_BIT5_Toggle=off  GPIO_Bit6=off  GPIO_BIT6_Toggle=off  GPIO_Bit7=on  GPIO_BIT7_Toggle=off
      settings: SourceProductBaseCode=TIC2000
  INV Enable : Constant  Value=0  OutDataTypeStr=uint16
  wires:
  INV Enable/1 -> Digital Output1/1

== system mcb_pmsm_foc_sensorless_hvkit_f28069m/Embedded Processor/Hardware Init/Offset Calculation/Code Generation/Default ADC Offset ==
  Constant : Constant  Value=inverter.CtSensAOffset  OutDataTypeStr=Inherit: Inherit via back propagation
  Constant1 : Constant  Value=inverter.CtSensBOffset  OutDataTypeStr=Inherit: Inherit via back propagation
  Data Store Write1 : DataStoreWrite  DataStoreName=IaOffset  IndexOptions=Index vector (dialog)  Indices=1  OutputSizes=1
  Data Store Write2 : DataStoreWrite  DataStoreName=IbOffset  IndexOptions=Index vector (dialog)  Indices=1  OutputSizes=1
  wires:
  Constant/1 -> Data Store Write1/1
  Constant1/1 -> Data Store Write2/1
